simulink model "detector"  (R2020b)
settings: Solver=VariableStepAuto  StartTime=0.0  StopTime=100  RelTol=1e-3
libraries: simulink x1
settings Model: Creator=Bk_space  LastModifiedBy=Bk_space

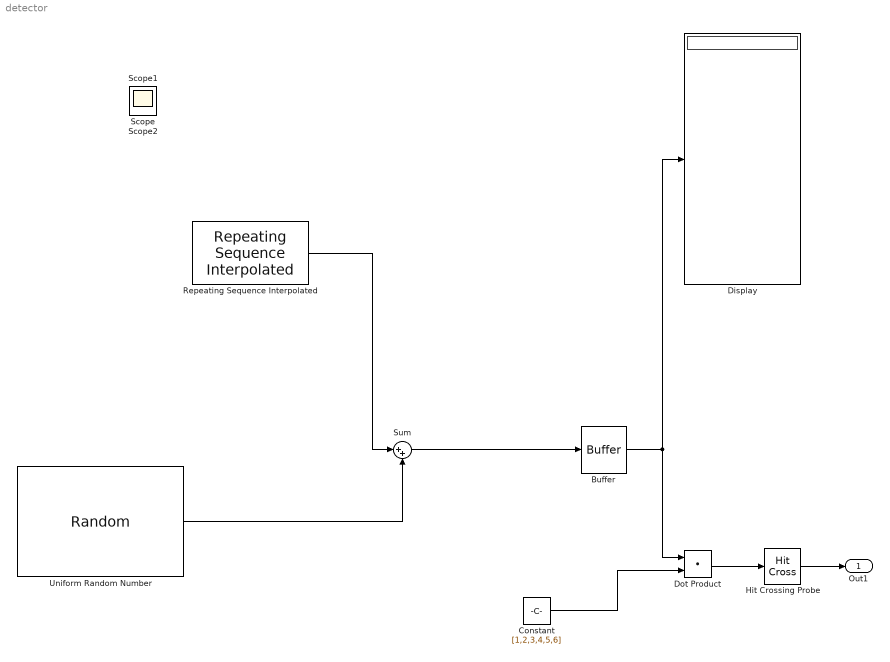
== system detector ==
  Buffer : Buffer  N=6  V=5  OutputFrames=off
  Constant : Constant  Value=[1,2,3,4,5,6]  SampleTime=0.1
  Display : Display
  Dot Product : DotProduct  InputSameDT=on  OutDataTypeStr=Inherit: Inherit via internal rule
  Hit Crossing Probe : HitCross  HitCrossingOffset=15  HitCrossingDirection=rising
  Repeating Sequence Interpolated : simulink/Sources/Repeating Sequence Interpolated  OutValues=TRAINGLE  TimeValues=TIMESTAMP  LookUpMeth=Interpolation-Use End Values  tsamp=0.01  OutMin=[]  OutMax=[]  OutDataTypeStr=double  OutputDataTypeScalingMode=double  OutDataType=fixdt(0,8)  OutScaling=2^-10
  Sum : Sum  Inputs=|++
  Uniform Random Number : UniformRandomNumber  Minimum=0  Maximum=0.5  SampleTime=0.1
  Out1 : Outport
  Scope : Scope
  Scope1 : Scope
  Scope2 : Scope
  wires:
  Uniform Random Number/1 -> Sum/2
  Sum/1 -> Buffer/1
  Repeating Sequence Interpolated/1 -> Sum/1
  Buffer/1 -> Display/1, Dot Product/1
  Constant/1 -> Dot Product/2
  Dot Product/1 -> Hit Crossing Probe/1
  Hit Crossing Probe/1 -> Out1/1
